simulink model "q19c"  (R2016a)
settings: Solver=VariableStepAuto  StartTime=0.0  StopTime=10.0  RelTol=1e-3
settings Model: Creator=Satya  LastModifiedBy=Satya

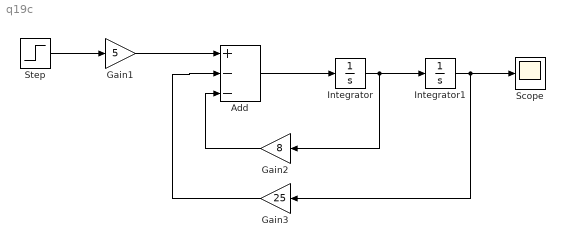
== system q19c ==
  Add : Sum  Inputs=+--
  Gain1 : Gain  Gain=5
  Gain2 : Gain  Gain=8
  Gain3 : Gain  Gain=25
  Integrator : Integrator
  Integrator1 : Integrator
  Scope : Scope
  Step : Step  SampleTime=0
  wires:
  Integrator/1 -> Gain2/1, Integrator1/1
  Integrator1/1 -> Gain3/1, Scope/1
  Add/1 -> Integrator/1
  Step/1 -> Gain1/1
  Gain1/1 -> Add/1
  Gain2/1 -> Add/3
  Gain3/1 -> Add/2
